simulink model "Example1_Connecting_To_The_AR_Drone"  (R2016a)
settings: configuration reference "AR_Drone_ConfigSet" (kept outside this file)
libraries: AR_Drone_Actuators x2, AR_Drone_Sensors x1
settings Model: SimulationMode=external  Creator=sannem  LastModifiedBy=sannem
settings ConfigSetRef: SourceLocation=Base Workspace

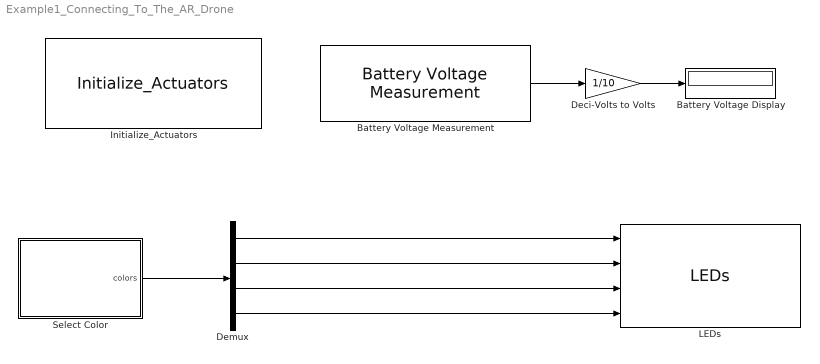
== system Example1_Connecting_To_The_AR_Drone ==
  Battery Voltage Display : Display
  Battery Voltage Measurement : AR_Drone_Sensors/Battery Voltage Measurement  SFunctionSpec=void BatteryMeasure_step(single y1[1])  SampleTime=-1
  Deci-Volts to Volts : Gain  Gain=1/10
  Demux : Demux
  Initialize_Actuators : AR_Drone_Actuators/Initialize_Actuators  ShowSpec=on
  LEDs : AR_Drone_Actuators/LEDs
  Select Color : MATLAB Function  TreatAsAtomicUnit=on  SystemSampleTime=1/2  mask(Color selector){input=Random}
      mask prompts: input "Select LED color"
      mask help: Use the drop down menu to select the color of the LEDs
  wires:
  Select Color/1(colors) -> Demux/1
  Demux/2 -> LEDs/2
  Demux/3 -> LEDs/3
  Demux/1 -> LEDs/1
  Demux/4 -> LEDs/4
  Deci-Volts to Volts/1 -> Battery Voltage Display/1
  Battery Voltage Measurement/1 -> Deci-Volts to Volts/1

== matlab function Example1_Connecting_To_The_AR_Drone/Select Color ==
  data: colors output; input parameter
function colors = ColorSelector(input)

outColors = [0 0 0 0];

switch input
    case 1
        outColors = [0 0 0 0];
    case 2
        outColors = [3 3 3 3];
    case 3
        outColors = [1 1 1 1];
    case 4
        outColors = [2 2 2 2];
    case 5
        outColors = floor(4 * rand(1,4));
    otherwise
        outColors = [0 0 0 0];
end
colors = outColors;
end
